simulink library "ESA_L2"  (R2024b)
settings: Solver=VariableStepAuto  StartTime=0.0  StopTime=10.0  RelTol=1e-3

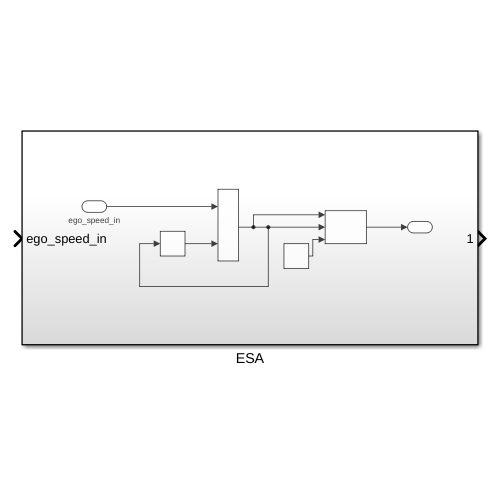
[thumbnail: Simulink's stored preview of the top-level diagram]
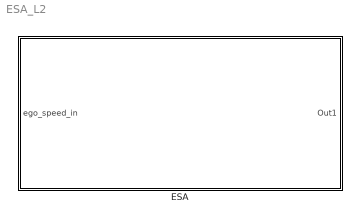
== system ESA_L2 ==
  ESA : Subsystem

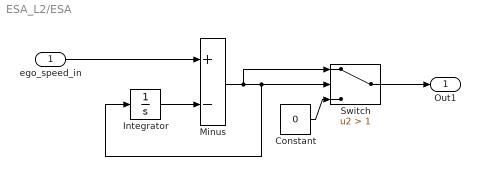
== system ESA_L2/ESA ==
  ego_speed_in : Inport
  Constant : Constant  Value=0
  Integrator : Integrator
  Minus : Sum  Inputs=+-
  Switch : Switch  Criteria=u2 > Threshold  Threshold=1  SaturateOnIntegerOverflow=off  InputSameDT=off
  Out1 : Outport
  wires:
  ego_speed_in/1 -> Minus/1
  Integrator/1 -> Minus/2
  Constant/1 -> Switch/3
  Switch/1 -> Out1/1
  Minus/1 -> Switch/1, Integrator/1, Switch/2
